simulink model "BuckBoost"  (R2018a)
settings: Solver=FixedStepDiscrete  StartTime=0.0  StopTime=5e-2  FixedStep=sampling_time  RelTol=1e-3
values from neighbouring files (symbols this model uses):
  C = 100e-6    (= 0.0001)    [sim_param.m]
  D = 0.75    [sim_param.m]
  f_s = 100e3    (= 100000)    [sim_param.m]
  L = 10e-6    (= 1e-05)    [sim_param.m]
  R_Load = 8    [sim_param.m]
  sampling_time = 1e-8    (= 1e-08)    [sim_param.m]
  V_d = 8.5    [sim_param.m]
libraries: powerlib x15, powerlib_meascontrol x1, pePwmGenerator x1
settings Model: Creator=enes_  LastModifiedBy=enes_

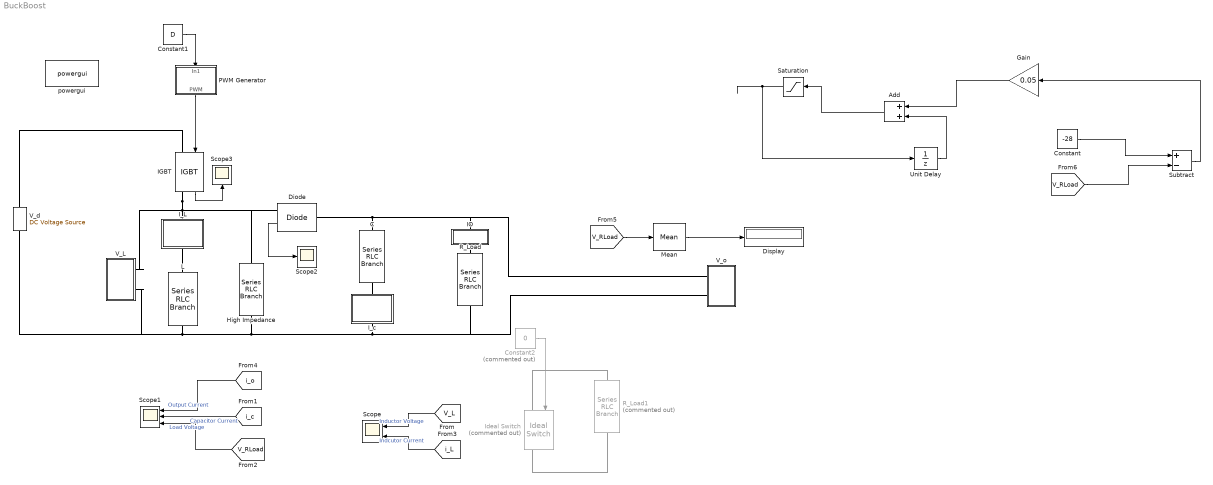
== system BuckBoost ==
  Add : Sum
  C : powerlib/Elements/Series RLC Branch  LConnTagsString=__new0  RConnTagsString=__new0  BranchType=C  Resistance=1  Inductance=L  SetiL0=off  InitialCurrent=0  Capacitance=C  Setx0=off  InitialVoltage=0  Measurements=None
  Constant : Constant  Value=-28
  Constant1 : Constant  Value=D
  Constant2 : Constant  Commented=on  Value=0
  Diode : powerlib/Power Electronics/Diode  Ron=1e-6  Lon=0  Vf=0  IC=0  UseSnubber=0  Rs=inf  Cs=0  Measurements=on
  Display : Display
  Gain : Gain  Gain=0.05
  High Impedance : powerlib/Elements/Series RLC Branch  LConnTagsString=__new0  RConnTagsString=__new0  BranchType=R  Resistance=1e9  Inductance=L  SetiL0=off  InitialCurrent=0  Capacitance=C  Setx0=off  InitialVoltage=0  Measurements=None
  IGBT : powerlib/Power Electronics/IGBT  Ron=1e-7  Lon=0  Vf=0  Tf=1e-6  Tt=2e-6  IC=0  Rs=inf  Cs=0  Measurements=on
  IO : Subsystem
  I_L : Subsystem
  I_c : Subsystem
  Ideal Switch : powerlib/Power Electronics/Ideal Switch  Commented=on  Ron=0.001  Lon=0  IC=1  Rs=1e5  Cs=inf  Measurements=on
  L : powerlib/Elements/Series RLC Branch  LConnTagsString=__new0  RConnTagsString=__new0  BranchType=RL  Resistance=1e-2  Inductance=L  SetiL0=off  InitialCurrent=0  Capacitance=1e-6  Setx0=off  InitialVoltage=0  Measurements=None
  Mean : powerlib_meascontrol/Measurements/Mean  Freq=1e5  Vinit=0  Ts=1e-8
  PWM Generator : Subsystem
  R_Load : powerlib/Elements/Series RLC Branch  LConnTagsString=__new0  RConnTagsString=__new0  BranchType=R  Resistance=R_Load  Inductance=L  SetiL0=off  InitialCurrent=0  Capacitance=C  Setx0=off  InitialVoltage=0  Measurements=None
  R_Load1 : powerlib/Elements/Series RLC Branch  Commented=on  LConnTagsString=__new0  RConnTagsString=__new0  BranchType=R  Resistance=72  Inductance=L  SetiL0=off  InitialCurrent=0  Capacitance=C  Setx0=off  InitialVoltage=0  Measurements=None
  Saturation : Saturate  UpperLimit=0.8  LowerLimit=0.1
  Scope : Scope  NumInputPorts=2
  Scope1 : Scope  NumInputPorts=3
  Scope2 : Scope
  Scope3 : Scope
  Subtract : Sum  Inputs=+-
  Unit Delay : UnitDelay  SampleTime=-1
  V_L : Subsystem
  V_d : powerlib/Electrical Sources/DC Voltage Source  Amplitude=V_d  Measurements=None
  V_o : Subsystem
  powergui : powerlib/powergui  Priority=1  SimulationMode=Discrete  SampleTime=sampling_time  frequency=60  Iterations=50  frequencyindice=0  Pbase=100e6  ErrMax=1e-4  UnitsV=kV  UnitsW=MW  buscounter=0  FunctionMessages=off  echomessages=off  EnableUseOfTLC=off  CurrentSourceSwitches=off  DisableSnubberDevices=off  DisableRonSwitches=off  DisableVfSwitches=off  DisplayEquations=off  SolverType=Tustin/Backward Euler (TBE)  Interpol=off  ExternalGateDelay=off  methode=off  Ts=100  x0status=blocks  SPID=on  SwTol=0  HookPort=off  RestoreLinks=warning  ResistiveCurrentMeasurement=off  Frange=[0:2:500]  Ylog=off  Xlog=on  ShowGrid=off  save=off  variable=ZData  structure=Diode  ZoomFFT=off  StartTime=0.02  cycles=100  DisplayStyle=6  fundamental=100e3  FreqAxis=off  MaxFrequency=1e7  frequencyindicesteady=1  RmsSteady=1  display=off
  wires:
  PWM Generator/1(PWM) -> IGBT/1
  [V_L] -> Scope/1  "Inductor Voltage"
  [i_L] -> Scope/2  "Indcutor Current"
  [i_o] -> Scope1/1  "Output Current"
  [i_c] -> Scope1/2  "Capacitor Current"
  [V_RLoad] -> Scope1/3  "Load Voltage"
  Diode/1 -> Scope2/1
  IGBT/1 -> Scope3/1
  [V_RLoad] -> Mean/1
  Mean/1 -> Display/1
  Constant/1 -> Subtract/1
  Gain/1 -> Add/1
  Unit Delay/1 -> Add/2
  Subtract/1 -> Gain/1
  [V_RLoad] -> Subtract/2
  Add/1 -> Saturation/1
  Saturation/1 -> Unit Delay/1
  Constant1/1 -> PWM Generator/1(In1)
  Constant2/1 -> Ideal Switch/1
  connections:
  V_d/RConn1 -- IGBT/LConn1
  IGBT/RConn1 -- High Impedance/RConn1 -- Diode/RConn1 -- V_L/LConn1 -- I_L/LConn1
  L/RConn1 -- High Impedance/LConn1 -- R_Load/RConn1 -- V_o/LConn2 -- I_c/LConn1 -- V_L/LConn2 -- V_d/LConn1
  C/LConn1 -- IO/LConn1 -- V_o/LConn1 -- Diode/LConn1
  I_c/RConn1 -- C/RConn1
  L/LConn1 -- I_L/RConn1
  IO/RConn1 -- R_Load/LConn1
  R_Load1/LConn1 -- Ideal Switch/LConn1
  Ideal Switch/RConn1 -- R_Load1/RConn1

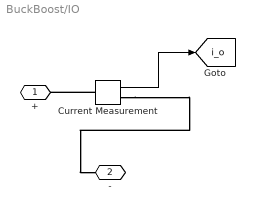
== system BuckBoost/IO ==
  Current Measurement : powerlib/Measurements/Current Measurement  PhasorSimulation=off  OutputType=Complex  PSBequivalent=0
  + : PMIOPort  Side=Left
  - : PMIOPort  Port=2  Side=Right
  tag scope: i_o=global
  wires:
  Current Measurement/1 -> [i_o]
  connections:
  Current Measurement/LConn1 -- +/RConn1
  Current Measurement/RConn1 -- -/RConn1

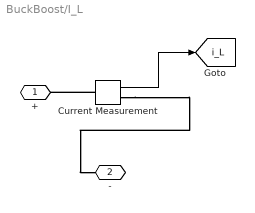
== system BuckBoost/I_L ==
  Current Measurement : powerlib/Measurements/Current Measurement  PhasorSimulation=off  OutputType=Complex  PSBequivalent=0
  + : PMIOPort  Side=Left
  - : PMIOPort  Port=2  Side=Right
  tag scope: i_L=global
  wires:
  Current Measurement/1 -> [i_L]
  connections:
  Current Measurement/LConn1 -- +/RConn1
  Current Measurement/RConn1 -- -/RConn1

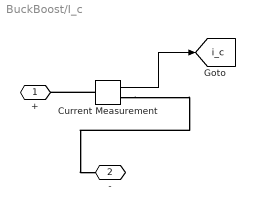
== system BuckBoost/I_c ==
  Current Measurement : powerlib/Measurements/Current Measurement  PhasorSimulation=off  OutputType=Complex  PSBequivalent=0
  + : PMIOPort  Side=Left
  - : PMIOPort  Port=2  Side=Right
  tag scope: i_c=global
  wires:
  Current Measurement/1 -> [i_c]
  connections:
  Current Measurement/LConn1 -- +/RConn1
  Current Measurement/RConn1 -- -/RConn1

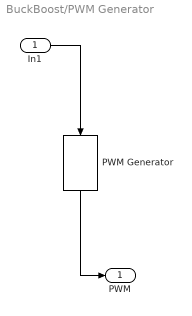
== system BuckBoost/PWM Generator ==
  In1 : Inport
  PWM Generator : pePwmGenerator/PWM Generator  CarrCount=Up  Tper=1/f_s  Ts=sampling_time
  PWM : Outport
  wires:
  In1/1 -> PWM Generator/1
  PWM Generator/1 -> PWM/1

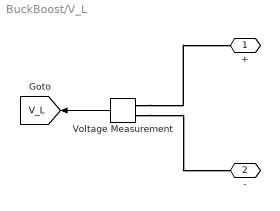
== system BuckBoost/V_L ==
  Voltage Measurement : powerlib/Measurements/Voltage Measurement  PhasorSimulation=off  OutputType=Complex  PSBequivalent=0
  + : PMIOPort  Side=Left
  - : PMIOPort  Port=2  Side=Left
  tag scope: V_L=global
  wires:
  Voltage Measurement/1 -> [V_L]
  connections:
  Voltage Measurement/LConn2 -- -/RConn1
  Voltage Measurement/LConn1 -- +/RConn1

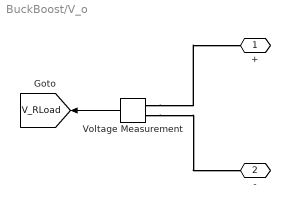
== system BuckBoost/V_o ==
  Voltage Measurement : powerlib/Measurements/Voltage Measurement  PhasorSimulation=off  OutputType=Complex  PSBequivalent=0
  + : PMIOPort  Side=Left
  - : PMIOPort  Port=2  Side=Left
  tag scope: V_RLoad=global
  wires:
  Voltage Measurement/1 -> [V_RLoad]
  connections:
  Voltage Measurement/LConn2 -- -/RConn1
  Voltage Measurement/LConn1 -- +/RConn1
